simulink library "Lib_HPF"  (R2021a)
settings: Solver=VariableStepAuto  StartTime=0.0  StopTime=10.0  RelTol=1e-3
settings Model: Creator=30610  LastModifiedBy=user

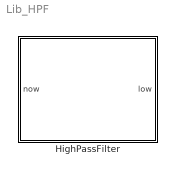
== system Lib_HPF ==
  HighPassFilter : Subsystem  mask{La=0, Lb=0}
      mask prompts: La "Gain_La"; Lb "Gain_Lb"
      mask DialogControl Container4 Prompt: HPF Discrete-time realization​
      mask DialogControl Control3 Prompt: y(n) = Laㆍy(n-1) + Lbㆍ(x(n)-x(n-1))
      mask DialogControl Control4 Prompt: La = (2-Tsw)/(2+Tsw)
      mask DialogControl Control5 Prompt: Lb = 2/(2+Tsw)
      mask DialogControl Container6 Prompt: High Pass Filter Gain

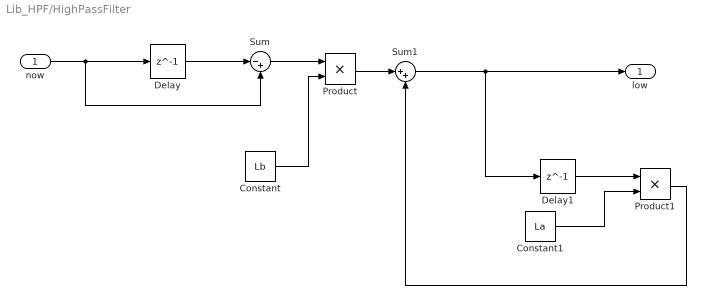
== system Lib_HPF/HighPassFilter ==
  now : Inport  OutDataTypeStr=single
  Constant : Constant  Value=Lb  OutDataTypeStr=single
  Constant1 : Constant  Value=La  OutDataTypeStr=single
  Delay : Delay  DelayLength=1  InitialCondition=0  StateName=HPF_Delta_old
  Delay1 : Delay  DelayLength=1  InitialCondition=0  StateName=HPF_Delta_low_z
  Product : Product
  Product1 : Product
  Sum : Sum  Inputs=|-+
  Sum1 : Sum  Inputs=|++
  low : Outport  OutDataTypeStr=single  VectorParamsAs1DForOutWhenUnconnected=off
  wires:
  Constant/1 -> Product/2
  Sum1/1 -> Delay1/1, low/1
  Product1/1 -> Sum1/2
  Delay1/1 -> Product1/1
  Product/1 -> Sum1/1
  now/1 -> Sum/2, Delay/1
  Sum/1 -> Product/1
  Delay/1 -> Sum/1
  Constant1/1 -> Product1/2
